simulink model "PD_discrete"  (R2016b)
settings: Solver=VariableStepAuto  StartTime=0.0  StopTime=10.0  RelTol=1e-3
values from neighbouring files (symbols this model uses):
  down = -up    (= -0.0872664625997)    [PD.m]    (also in PD_statespace_discrete.m)
  Ts = 0.02    [PD.m]    (also in PD_statespace_discrete.m)
  up = 5*pi/180    (= 0.0872664625997)    [PD.m]    (also in PD_statespace_discrete.m)
libraries: cstblocks x2
settings Model: Creator=Ashraf  LastModifiedBy=Ashraf

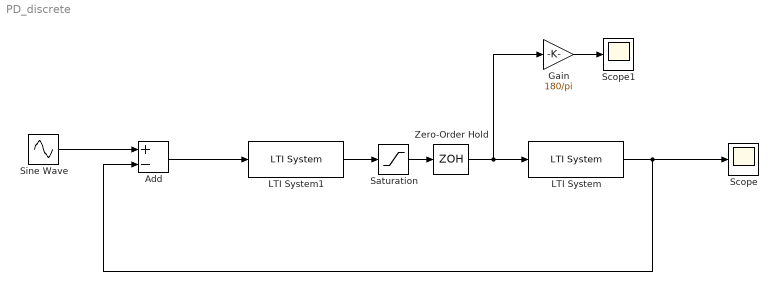
== system PD_discrete ==
  Add : Sum  Inputs=+-
  Gain : Gain  Gain=180/pi
  LTI System : cstblocks/LTI System  sys=X  IC=[]
  LTI System1 : cstblocks/LTI System  sys=C  IC=[]
  Saturation : Saturate  UpperLimit=up  LowerLimit=down
  Scope : Scope
  Scope1 : Scope
  Sine Wave : Sin  Amplitude=0.1  SampleTime=Ts
  Zero-Order Hold : ZeroOrderHold  SampleTime=Ts
  wires:
  LTI System1/1 -> Saturation/1
  Add/1 -> LTI System1/1
  Sine Wave/1 -> Add/1
  LTI System/1 -> Scope/1, Add/2
  Gain/1 -> Scope1/1
  Saturation/1 -> Zero-Order Hold/1
  Zero-Order Hold/1 -> Gain/1, LTI System/1
